simulink model "xiti4_5zhh_chqjzh001"  (Simulink 5.0)
settings: Solver=ode45  SolverMode=SingleTasking  StartTime=0.0  StopTime=1  FixedStep=0.1  RelTol=1e-3
settings Model: LastModifiedBy=ThinkPad

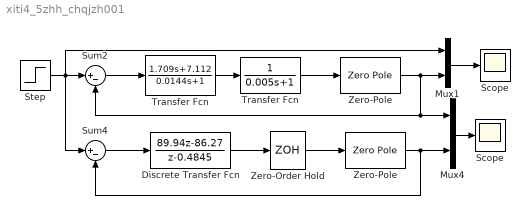
== system xiti4_5zhh_chqjzh001 ==
  "  Transfer Fcn " : TransferFcn  Denominator=[0.005 1]
  " Scope " : Scope
      settings: YMin=-3.5  YMax=1  SaveName=yyy  DataFormat=Array  MaxDataPoints=500000
  " Zero-Pole" : ZeroPole  Zeros=[]  Poles=[0 -1]  Gain=[10]
  "Discrete Transfer Fcn " : DiscreteTransferFcn  Numerator=[89.94 -86.27]  Denominator=[1 -0.4845]  SampleTime=0.01
  Mux1 : Mux  Inputs=2
  Mux4 : Mux  Inputs=2
  Scope : Scope
      settings: YMin=-3.5  YMax=1  MaxDataPoints=500000
  Step : Step  Time=0  SampleTime=0
  Sum2 : Sum  Inputs=|+-  SaturateOnIntegerOverflow=on
  Sum4 : Sum  Inputs=|+-  SaturateOnIntegerOverflow=on
  Transfer Fcn : TransferFcn  Numerator=[1.709 7.112]  Denominator=[0.0144 1]
  "Zero-Order Hold " : ZeroOrderHold  SampleTime=0.01
  "Zero-Pole " : ZeroPole  Zeros=[]  Poles=[0 -1]  Gain=[10]
  wires:
  Step/1 -> Sum2/1, Sum4/1, Mux1/1
  Mux4/1 -> " Scope "/1
  " Zero-Pole"/1 -> Mux4/2, Sum4/2
  "Discrete Transfer Fcn "/1 -> "Zero-Order Hold "/1
  Sum4/1 -> "Discrete Transfer Fcn "/1
  Mux1/1 -> Scope/1
  "Zero-Pole "/1 -> Mux1/2, Sum2/2, Mux4/1
  Transfer Fcn/1 -> "  Transfer Fcn "/1
  "  Transfer Fcn "/1 -> "Zero-Pole "/1
  Sum2/1 -> Transfer Fcn/1
  "Zero-Order Hold "/1 -> " Zero-Pole"/1
